simulink model "A3_reg_b"  (Simulink 7.0)
settings: Solver=ode45  StartTime=0.0  StopTime=80  MaxStep=.01  RelTol=1e-8
values from neighbouring files (symbols this model uses):
  F = 1/(C*(B*K-A)^-1 *B)    [Zugmaschine_Skript.m]
  f1 = 5    [Zugmaschine_Skript.m]
  f2 = 5    [Zugmaschine_Skript.m]
  K = place(A,B,P)    [Zugmaschine_Skript.m]
  m1 = .5    (= 0.5)    [Zugmaschine_Skript.m]
  m2 = 1    [Zugmaschine_Skript.m]
  m3 = 1    [Zugmaschine_Skript.m]
  x10 = 0    [Zugmaschine_Skript.m]
  x20 = 0    [Zugmaschine_Skript.m]
  x30 = 0    [Zugmaschine_Skript.m]
settings Model: Creator=Peter  LastModifiedBy=Peter

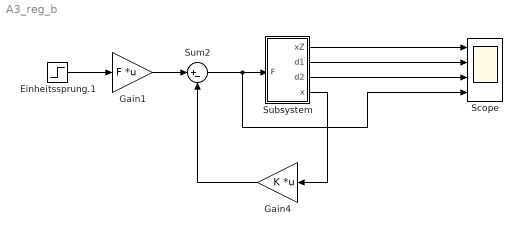
== system A3_reg_b ==
  Einheitssprung.1 : Step  Time=eps  After=100  SampleTime=0
  Gain1 : Gain  Gain=F  Multiplication=Matrix(K*u)  ParameterDataType=sfix(16)  ParameterScaling=2^0  OutDataType=sfix(16)  OutScaling=2^0
  Gain4 : Gain  Orientation=left  Gain=K  Multiplication=Matrix(K*u)  ParameterDataType=sfix(16)  ParameterScaling=2^0  OutDataType=sfix(16)  OutScaling=2^0
  Scope : Scope  NumInputPorts=4
      settings: TimeRange=100  YMin=0~-0.1~-0.06~-5  YMax=100~0.25~0.1~5
  Subsystem : Subsystem
  Sum2 : Sum  Inputs=|+-  OutDataType=sfix(16)  OutScaling=2^0
  wires:
  Sum2/1 -> Subsystem/1(F), Scope/4
  Subsystem/4(x) -> Gain4/1
  Gain4/1 -> Sum2/2
  Gain1/1 -> Sum2/1
  Einheitssprung.1/1 -> Gain1/1
  Subsystem/1(xZ) -> Scope/1
  Subsystem/2(d1) -> Scope/2
  Subsystem/3(d2) -> Scope/3

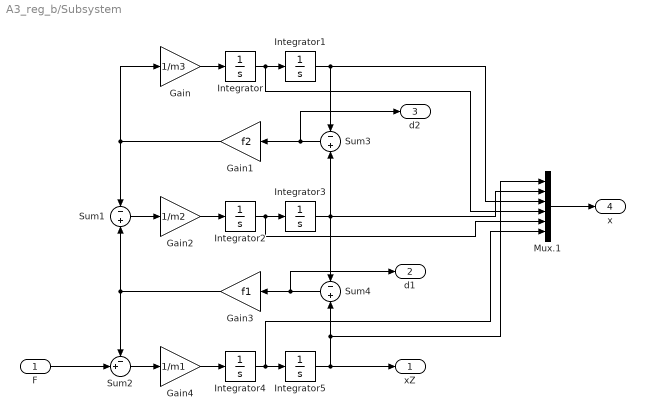
== system A3_reg_b/Subsystem ==
  F : Inport  OutDataType=sfix(16)  OutScaling=2^0
  Gain : Gain  Gain=1/m3  ParameterDataType=sfix(16)  ParameterScaling=2^0  OutDataType=sfix(16)  OutScaling=2^0
  Gain1 : Gain  Orientation=left  Gain=f2  ParameterDataType=sfix(16)  ParameterScaling=2^0  OutDataType=sfix(16)  OutScaling=2^0
  Gain2 : Gain  Gain=1/m2  ParameterDataType=sfix(16)  ParameterScaling=2^0  OutDataType=sfix(16)  OutScaling=2^0
  Gain3 : Gain  Orientation=left  Gain=f1  ParameterDataType=sfix(16)  ParameterScaling=2^0  OutDataType=sfix(16)  OutScaling=2^0
  Gain4 : Gain  Gain=1/m1  ParameterDataType=sfix(16)  ParameterScaling=2^0  OutDataType=sfix(16)  OutScaling=2^0
  Integrator : Integrator
  Integrator1 : Integrator  InitialCondition=x10
  Integrator2 : Integrator
  Integrator3 : Integrator  InitialCondition=x20
  Integrator4 : Integrator
  Integrator5 : Integrator  InitialCondition=x30
  Mux.1 : Mux  Inputs=6
  Sum1 : Sum  Inputs=-+  OutDataType=sfix(16)  OutScaling=2^0
  Sum2 : Sum  Inputs=-+|  OutDataType=sfix(16)  OutScaling=2^0
  Sum3 : Sum  Orientation=left  Inputs=-+  OutDataType=sfix(16)  OutScaling=2^0
  Sum4 : Sum  Orientation=left  Inputs=-+  OutDataType=sfix(16)  OutScaling=2^0
  xZ : Outport  OutDataType=sfix(16)  OutScaling=2^0
  d1 : Outport  Port=2  OutDataType=sfix(16)  OutScaling=2^0
  d2 : Outport  Port=3  OutDataType=sfix(16)  OutScaling=2^0
  x : Outport  Port=4  OutDataType=sfix(16)  OutScaling=2^0
  wires:
  Integrator/1 -> Integrator1/1, Mux.1/4
  Gain/1 -> Integrator/1
  Gain1/1 -> Gain/1, Sum1/1
  Integrator2/1 -> Integrator3/1, Mux.1/5
  Gain2/1 -> Integrator2/1
  Sum1/1 -> Gain2/1
  Integrator3/1 -> Sum4/1, Sum3/2, Mux.1/2
  Gain3/1 -> Sum2/1, Sum1/2
  Integrator4/1 -> Integrator5/1, Mux.1/6
  Gain4/1 -> Integrator4/1
  Sum2/1 -> Gain4/1
  Integrator5/1 -> xZ/1, Sum4/2, Mux.1/1
  Integrator1/1 -> Sum3/1, Mux.1/3
  Sum3/1 -> d2/1, Gain1/1
  Sum4/1 -> Gain3/1, d1/1
  F/1 -> Sum2/2
  Mux.1/1 -> x/1
